simulink model "untitled"  (Simulink 5.0)
settings: Solver=ode45  StartTime=0.0  StopTime=60  RelTol=1e-3
settings Model: LastModifiedBy=Imed

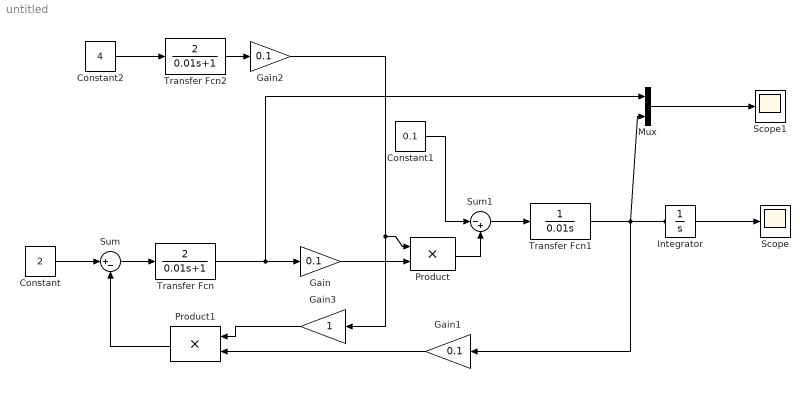
== system untitled ==
  Constant : Constant  Value=2
  Constant1 : Constant  Value=0.1
  Constant2 : Constant  Value=4
  Gain : Gain  Gain=0.1  SaturateOnIntegerOverflow=on
  Gain1 : Gain  Orientation=left  Gain=0.1  SaturateOnIntegerOverflow=on
  Gain2 : Gain  Gain=0.1  SaturateOnIntegerOverflow=on
  Gain3 : Gain  Orientation=left  SaturateOnIntegerOverflow=on
  Integrator : Integrator
  Mux : Mux  Inputs=2
  Product : Product  SaturateOnIntegerOverflow=on
  Product1 : Product  Orientation=left  SaturateOnIntegerOverflow=on
  Scope : Scope
  Scope1 : Scope
      settings: TimeRange=90  YMin=-2  YMax=12
  Sum : Sum  Inputs=|+-  SaturateOnIntegerOverflow=on
  Sum1 : Sum  Inputs=|-+  SaturateOnIntegerOverflow=on
  Transfer Fcn : TransferFcn  Numerator=[2]  Denominator=[0.01 1]
  Transfer Fcn1 : TransferFcn  Denominator=[0.01 0]
  Transfer Fcn2 : TransferFcn  Numerator=[2]  Denominator=[0.01 1]
  wires:
  Constant/1 -> Sum/1
  Sum/1 -> Transfer Fcn/1
  Constant1/1 -> Sum1/1
  Sum1/1 -> Transfer Fcn1/1
  Transfer Fcn1/1 -> Integrator/1, Mux/2, Gain1/1
  Integrator/1 -> Scope/1
  Mux/1 -> Scope1/1
  Product/1 -> Sum1/2
  Gain2/1 -> Product/1, Gain3/1
  Gain1/1 -> Product1/2
  Product1/1 -> Sum/2
  Gain/1 -> Product/2
  Transfer Fcn/1 -> Gain/1, Mux/1
  Gain3/1 -> Product1/1
  Transfer Fcn2/1 -> Gain2/1
  Constant2/1 -> Transfer Fcn2/1
